simulink model "Circulator"  (R2024b)
settings: Solver=VariableStepAuto  StartTime=0.0  StopTime=10.0  RelTol=1e-3
libraries: simrfV2util1 x3, simrfV2junction1 x1, simrfV2sources1 x1

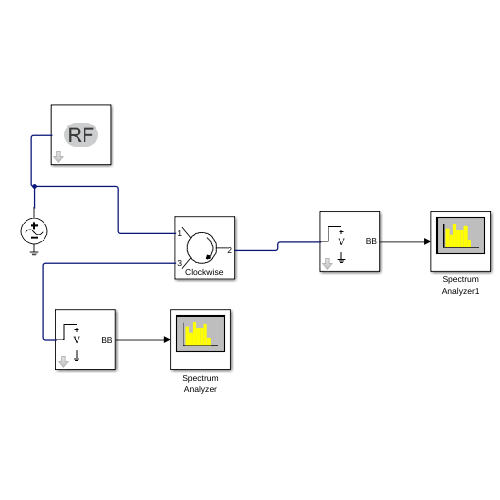
[thumbnail: Simulink's stored preview of the top-level diagram]
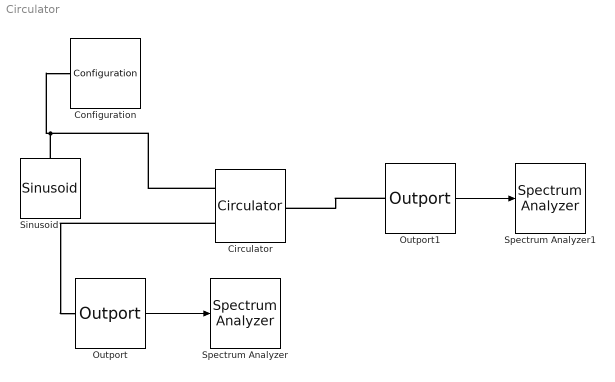
== system Circulator ==
  Circulator : simrfV2junction1/Circulator  classname=circulators  DataSource=Network-parameters  NumPorts=3  DeviceCirculator=Circulator clockwise  DeviceDivider=T power divider  DeviceCoupler=Directional coupler  Paramtype=S-parameters  Sparam=[0 0 1; 1 0 0; 0 1 0]  SparamFreq=1e9 Hz  SparamZ0=50  Phase12=0  Phase33=0  Alpha=0  NumberDividerOutports=2  Coupling=0  Directivity=inf  InsertionLoss=inf  ReturnLoss=inf  InternalGrounding=on  SparamRepresentation=Frequency domain  FitOpt=Share all poles  FitTol=-40  MaxPoles=48
  Configuration : simrfV2util1/Configuration  AutoFreq=on  Tones=[] Hz  Harmonics=[]  NormalizeCarrierPower=on  SolverType=Auto  UseCCode=on  StepSize=1e-6 s  AddNoise=on  defaultRNG=on  Seed=0  Temperature=290.0 K  SolverDelFlag=0  AbsTol=1e-6  RelTol=1e-3  MaxIter=10  ErrorEstimationType=2-norm over all variables  EnableInterpFilter=on  HiddenFIRfilterControllerParam=off  SmallSignalApprox=off  AllSimFreqs=on  SimFreqs=[] Hz  SimFreqsInternal=[]  SamplesPerFrame=1
  Outport : simrfV2util1/Outport  SensorType=Ideal voltage  OutputFormat=Complex Baseband  CarrierFreq=0 Hz  ZL=Inf  InternalGrounding=on  StepSize=1e-6 s  AutoStep=on  HalfPolyphaseLength=12
  Outport1 : simrfV2util1/Outport  SensorType=Ideal voltage  OutputFormat=Complex Baseband  CarrierFreq=0 Hz  ZL=Inf  InternalGrounding=on  StepSize=1e-6 s  AutoStep=on  HalfPolyphaseLength=12
  Sinusoid : simrfV2sources1/Sinusoid  SineSourceType=Ideal voltage  VO_I=0 V  IO_I=0 A  VO_Q=0 V  IO_Q=0 A  VA_I=1 V  IA_I=0 A  VA_Q=0 V  IA_Q=0 A  Fmod=1 GHz  TD=0 s  CarrierFreq=0 Hz  InternalGrounding=on
  Spectrum Analyzer : SpectrumAnalyzer  Tag=simrfV2util1/Spectrum Analyzer  WindowPosition=[918.400024,42.000000,541.000000,564.000000,]  Visible=on  ScopeFrameLocation=window  Method=Welch  AveragingMethod=Exponential  AllowFFTLengthLessThanSamplesPerUpdate=on
  Spectrum Analyzer1 : SpectrumAnalyzer  Tag=simrfV2util1/Spectrum Analyzer  WindowPosition=[209.400009,39.000000,560.000000,560.000000,]  Visible=on  ScopeFrameLocation=window  Method=Welch  AveragingMethod=Exponential  YLimits=[-198.80579611,-136.29640331]  AllowFFTLengthLessThanSamplesPerUpdate=on
  wires:
  Outport/1 -> Spectrum Analyzer/1
  Outport1/1 -> Spectrum Analyzer1/1
  connections:
  Circulator/LConn1 -- Sinusoid/LConn1 -- Configuration/LConn1
  Circulator/LConn2 -- Outport/LConn1
  Outport1/LConn1 -- Circulator/RConn1
